simulink model "Bicycle_CTRA"  (R2018a)
settings: Solver=ode45  StartTime=0.0  StopTime=60  FixedStep=0.1  MaxStep=0.05  MinStep=1e-5  RelTol=1e-6  EnableMultiTasking=on
StopFcn:
  | run('CTRA_plotter.m');
model workspace (MAT data in the model file):
  B = 1.5289
  C = 1.0901
  D = 0.6
  E = -0.95084
  Iw = 1
  Iz = 1700
  Kphi_f = 57
  Kphi_r = 57
  hrc_f = 0
  hrc_r = 0
  hs = 0.56
  lf = 1
  lr = 1.6
  m = 1200
  re = 0.32
  tr = 1.5
undefined symbols (not defined in the file or in its folder): sigbuilder_block
libraries: commchan3 x6, simulink x1
settings Model: Creator=michaelstolz  LastModifiedBy=Mora
settings SolverCC: ZeroCrossControl=EnableAll  AutoInsertRateTranBlk=on  InsertRTBMode=Always
settings DataIOCC: SaveFormat=StructureWithTime  SignalLoggingSaveFormat=ModelDataLogs  SaveOutput=off  SignalLogging=off  SaveTime=off
settings OptimizationCC: LifeSpan=inf
settings DebuggingCC: UnderspecifiedInitializationDetection=Classic  MergeDetectMultiDrivingBlocksExec=none  SolverPrmCheckMsg=warning  FcnCallInpInsideContextMsg=warning  SFUnexpectedBacktrackingDiag=warning  SFNoUnconditionalDefaultTransitionDiag=warning  SFExecutionAtInitializationDiag=none
settings HardwareCC: ProdBitPerPointer=32  ProdBitPerSizeT=32  ProdBitPerPtrDiffT=32  ProdLargestAtomicFloat=None  ProdIntDivRoundTo=Undefined  ProdEndianess=Unspecified  ProdWordSize=32  ProdHWDeviceType=32-bit Generic
settings ModelReferenceCC: PropagateSignalLabelsOutOfModel=off
settings SFSimCC: SimParseCustomCode=off
settings CodeAppCC: StateflowObjectComments=on
settings GRTTargetCC: TargetLangStandard=C89/C90 (ANSI)  GeneratePreprocessorConditionals=Disable all
settings ConfigComp: CovMetricSettings=dw  CovHtmlReporting=on  CovSaveCumulativeToWorkspaceVar=on  CovSaveSingleToWorkspaceVar=on  CovExternalEMLEnable=off

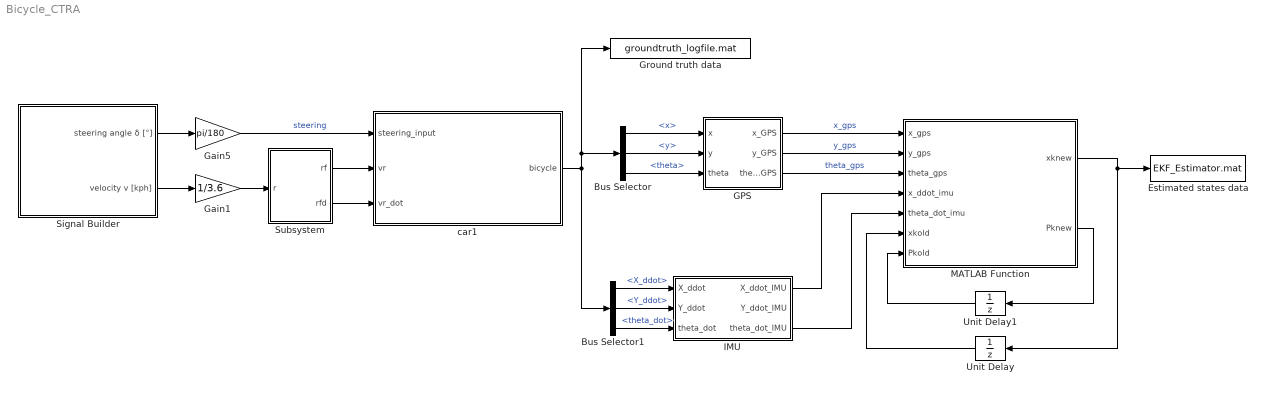
== system Bicycle_CTRA ==
  Bus Selector : BusSelector  OutputSignals=x,y,theta
  Bus Selector1 : BusSelector  OutputSignals=X_ddot,Y_ddot,theta_dot
  Estimated states data : ToFile  Filename=EKF_Estimator.mat  MatrixName=EKF  SaveFormat=Timeseries  SampleTime=1/50
  GPS : Subsystem
  Gain1 : Gain  Gain=1/3.6
  Gain5 : Gain  Gain=pi/180
  Ground truth data : ToFile  Filename=groundtruth_logfile.mat  MatrixName=GNDT  SaveFormat=Timeseries  SampleTime=1/50
  IMU : Subsystem
  MATLAB Function : MATLAB Function  TreatAsAtomicUnit=on
  Signal Builder : Subsystem  Tag=STV Subsys  LoadFcn=sigbuilder_block('load');  StartFcn=sigbuilder_block('start');  StopFcn=sigbuilder_block('stop');  ClipboardFcn=sigbuilder_block('clipboard');  mask(Sigbuilder block){tuvar=[0:10]}
      mask help: Simulink:masks:SigbuilderBlock_MD
      mask init:
      | if ~strcmp(get_param(bdroot(gcbh),'SimulationStatus'),'stopped') tuvar = sigbuilder_block('maskInit'); end
      settings: CopyFcn=sigbuilder_block('copy');  DeleteFcn=sigbuilder_block('delete');  ModelCloseFcn=sigbuilder_block('modelClose');  PreSaveFcn=sigbuilder_block('preSave');  PauseFcn=sigbuilder_block('pause');  ContinueFcn=sigbuilder_block('continue');  NameChangeFcn=sigbuilder_block('namechange');  OpenFcn=sigbuilder_block('open',[9 6 942 506.25 ]);  CloseFcn=sigbuilder_block('close');
      mask Display: plot(0, 0, 100, 100,[2, 2, 32, 32, 2], [68, 8, 8, 68, 68],[32, 2], [38, 38], [32, 19, 2],[53, 60, 44], [32, 17, 17, 2],[16, 16, 31, 31]);txt = getActiveGroup(gcbh);text(2, 100, txt,'verticalAlignment', 'top');
  Subsystem : Subsystem
  Unit Delay : UnitDelay  InitialCondition=[0, 0, 0.1, 1, 0.1, 0]'  SampleTime=-1
  Unit Delay1 : UnitDelay  InitialCondition=diag([1000000, 1000000, 10, 10, 10, 10],0)  SampleTime=-1
  car1 : Subsystem
  wires:
  Signal Builder/1(steering angle δ [°]) -> Gain5/1
  Signal Builder/2(velocity v [kph]) -> Gain1/1
  Gain5/1 -> car1/1(steering_input)  "steering"
  Subsystem/1(rf) -> car1/2(vr)
  car1/1(bicycle) -> Ground truth data/1, Bus Selector/1, Bus Selector1/1
  Bus Selector/1 -> GPS/1(x)  "<x>"
  Bus Selector/2 -> GPS/2(y)  "<y>"
  Gain1/1 -> Subsystem/1(r)
  Bus Selector/3 -> GPS/3(theta)  "<theta>"
  Subsystem/2(rfd) -> car1/3(vr_dot)
  Bus Selector1/1 -> IMU/1(X_ddot)  "<X_ddot>"
  Bus Selector1/2 -> IMU/2(Y_ddot)  "<Y_ddot>"
  Bus Selector1/3 -> IMU/3(theta_dot)  "<theta_dot>"
  GPS/1(x_GPS) -> MATLAB Function/1(x_gps)  "x_gps"
  GPS/2(y_GPS) -> MATLAB Function/2(y_gps)  "y_gps"
  GPS/3(theta_GPS) -> MATLAB Function/3(theta_gps)  "theta_gps"
  IMU/3(theta_dot_IMU) -> MATLAB Function/5(theta_dot_imu)
  MATLAB Function/2(Pknew) -> Unit Delay1/1
  MATLAB Function/1(xknew) -> Unit Delay/1, Estimated states data/1
  Unit Delay1/1 -> MATLAB Function/7(Pkold)
  Unit Delay/1 -> MATLAB Function/6(xkold)
  IMU/1(X_ddot_IMU) -> MATLAB Function/4(x_ddot_imu)

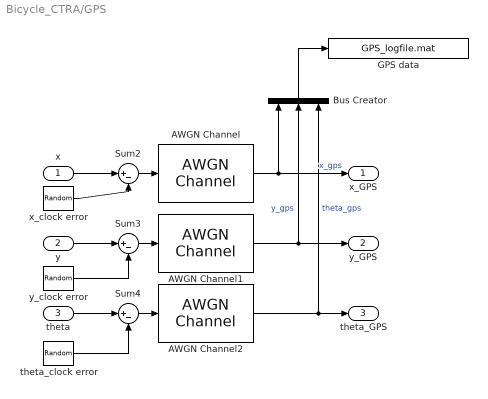
== system Bicycle_CTRA/GPS ==
  x : Inport
  y : Inport  Port=2
  theta : Inport  Port=3
  AWGN Channel : commchan3/AWGN Channel  InputProcessing=Columns as channels (frame based)  seed=40  noiseMode=Variance from mask  EbNodB=10  EsNodB=10  SNRdB=10  bitsPerSym=1  Ps=1  Tsym=1  variance=3
  AWGN Channel1 : commchan3/AWGN Channel  InputProcessing=Columns as channels (frame based)  seed=67  noiseMode=Variance from mask  EbNodB=10  EsNodB=10  SNRdB=10  bitsPerSym=1  Ps=1  Tsym=1  variance=3
  AWGN Channel2 : commchan3/AWGN Channel  InputProcessing=Columns as channels (frame based)  seed=67  noiseMode=Variance from mask  EbNodB=10  EsNodB=10  SNRdB=10  bitsPerSym=1  Ps=1  Tsym=1  variance=3/500
  Bus Creator : BusCreator  Inputs=3
  GPS data : ToFile  Filename=GPS_logfile.mat  MatrixName=GPS  SaveFormat=Timeseries  SampleTime=1/50
  Sum2 : Sum  Inputs=|+-
  Sum3 : Sum  Inputs=|+-
  Sum4 : Sum  Inputs=|+-
  theta_clock error : UniformRandomNumber  Minimum=0  Maximum=1e-9  SampleTime=3
  x_clock error : UniformRandomNumber  Minimum=0  Maximum=1e-9  SampleTime=3
  y_clock error : UniformRandomNumber  Minimum=0  Maximum=1e-9  SampleTime=3
  x_GPS : Outport
  y_GPS : Outport  Port=2
  theta_GPS : Outport  Port=3
  wires:
  AWGN Channel2/1 -> Bus Creator/3, theta_GPS/1  "theta_gps"
  x/1 -> Sum2/1
  Sum2/1 -> AWGN Channel/1
  Sum3/1 -> AWGN Channel1/1
  Sum4/1 -> AWGN Channel2/1
  y/1 -> Sum3/1
  y_clock error/1 -> Sum3/2
  AWGN Channel/1 -> Bus Creator/1, x_GPS/1  "x_gps"
  theta/1 -> Sum4/1
  AWGN Channel1/1 -> Bus Creator/2, y_GPS/1  "y_gps"
  x_clock error/1 -> Sum2/2
  theta_clock error/1 -> Sum4/2
  Bus Creator/1 -> GPS data/1

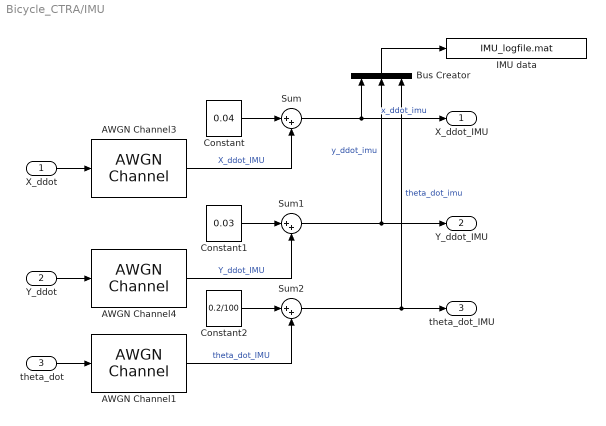
== system Bicycle_CTRA/IMU ==
  X_ddot : Inport
  Y_ddot : Inport  Port=2
  theta_dot : Inport  Port=3
  AWGN Channel1 : commchan3/AWGN Channel  InputProcessing=Columns as channels (frame based)  seed=67  noiseMode=Variance from mask  EbNodB=10  EsNodB=10  SNRdB=10  bitsPerSym=1  Ps=1  Tsym=1  variance=1/100
  AWGN Channel3 : commchan3/AWGN Channel  InputProcessing=Columns as channels (frame based)  seed=67  noiseMode=Variance from mask  EbNodB=10  EsNodB=10  SNRdB=10  bitsPerSym=1  Ps=1  Tsym=1  variance=0.08
  AWGN Channel4 : commchan3/AWGN Channel  InputProcessing=Columns as channels (frame based)  seed=67  noiseMode=Variance from mask  EbNodB=10  EsNodB=10  SNRdB=10  bitsPerSym=1  Ps=1  Tsym=1  variance=0.03
  Bus Creator : BusCreator  Inputs=3
  Constant : Constant  Value=0.04
  Constant1 : Constant  Value=0.03
  Constant2 : Constant  Value=0.2/100
  IMU data : ToFile  Filename=IMU_logfile.mat  MatrixName=IMU  SaveFormat=Timeseries  SampleTime=1/50
  Sum : Sum  Inputs=|++
  Sum1 : Sum  Inputs=|++
  Sum2 : Sum  Inputs=|++
  X_ddot_IMU : Outport
  Y_ddot_IMU : Outport  Port=2
  theta_dot_IMU : Outport  Port=3
  wires:
  X_ddot/1 -> AWGN Channel3/1
  Y_ddot/1 -> AWGN Channel4/1
  theta_dot/1 -> AWGN Channel1/1
  AWGN Channel3/1 -> Sum/2  "X_ddot_IMU"
  Sum/1 -> Bus Creator/1, X_ddot_IMU/1  "x_ddot_imu"
  Constant/1 -> Sum/1
  Constant1/1 -> Sum1/1
  Sum1/1 -> Bus Creator/2, Y_ddot_IMU/1  "y_ddot_imu"
  AWGN Channel4/1 -> Sum1/2  "Y_ddot_IMU"
  Constant2/1 -> Sum2/1
  Sum2/1 -> Bus Creator/3, theta_dot_IMU/1  "theta_dot_imu"
  AWGN Channel1/1 -> Sum2/2  "theta_dot_IMU"
  Bus Creator/1 -> IMU data/1

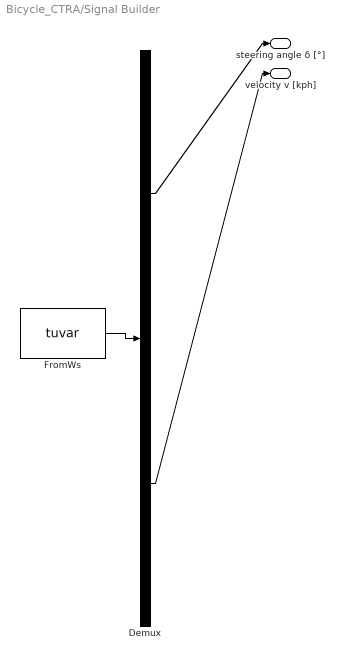
== system Bicycle_CTRA/Signal Builder ==
  Demux : Demux  Tag=STV Demux  Outputs=2
  FromWs : FromWorkspace  Tag=STV FromWs  VariableName=tuvar  SampleTime=0
      SigBuilderData=|
      | common.afterFinalStr = 'Extrapolate'
      | common.sampleTime = 0
      | dataSet(1).timeRange = [0 20]
      | dataSet(1).name = 'Line'
      | dataSet(2).timeRange = [0 20]
      | dataSet(2).name = 'Left curve'
      | dataSet(3).timeRange = [0 60]
      | dataSet(3).name = 'Line Curves'
      | sbobj.Groups(1).Name = 'Line'
      | sbobj.Groups(1).Signals(1).Name = 'steering angle δ [°]'
      | sbobj.Groups(1).Signals(1).XData = [0 20]
      | sbobj.Groups(1).Signals(1).YData = [0 0]
      | sbobj.Groups(1).Signals(2).Name = 'velocity v [kph]'
      | sbobj.Groups(1).Signals(2).XData = [0 6 15 20]
      | sbobj.Groups(1).Signals(2).YData = [0 100 150 150]
      | sbobj.Groups(1).TimeRange = [0 20]
      | sbobj.Groups(2).Name = 'Left curve'
      | sbobj.Groups(2).Signals(1).Name = 'steering angle δ [°]'
      | sbobj.Groups(2).Signals(1).XData = [0 20]
      | sbobj.Groups(2).Signals(1).YData = [3.61 3.61]
      | sbobj.Groups(2).Signals(2).Name = 'velocity v [kph]'
      | sbobj.Groups(2).Signals(2).XData = [0 10 20]
      | sbobj.Groups(2).Signals(2).YData = [0 79.5 80]
      | sbobj.Groups(2).TimeRange = [0 20]
      | sbobj.Groups(3).Name = 'Line Curves'
      | sbobj.Groups(3).Signals(1).Name = 'steering angle δ [°]'
      | sbobj.Groups(3).Signals(1).XData = [0 15 25 30 40 40 52 54 60]
      | sbobj.Groups(3).Signals(1).YData = [0 0 -2 -2 2 1.98 2 0 0]
      | sbobj.Groups(3).Signals(2).Name = 'velocity v [kph]'
      | sbobj.Groups(3).Signals(2).XData = [0 15 30 35 40 50 60]
      | sbobj.Groups(3).Signals(2).YData = [0 100 60 40 60 60 60]
      | sbobj.Groups(3).TimeRange = [0 60]
  steering angle δ [°] : Outport  Tag=STV Outport
  velocity v [kph] : Outport  Tag=STV Outport  Port=2
  wires:
  FromWs/1 -> Demux/1
  Demux/1 -> steering angle δ [°]/1
  Demux/2 -> velocity v [kph]/1

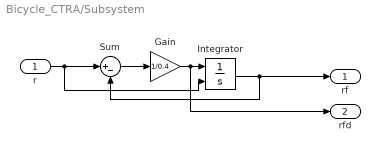
== system Bicycle_CTRA/Subsystem ==
  r : Inport
  Gain : Gain  Gain=1/0.4
  Integrator : Integrator  InitialConditionSource=external
  Sum : Sum  Inputs=|+-
  rf : Outport
  rfd : Outport  Port=2
  wires:
  Gain/1 -> rfd/1, Integrator/1
  Sum/1 -> Gain/1
  Integrator/1 -> rf/1, Sum/2
  r/1 -> Integrator/2, Sum/1

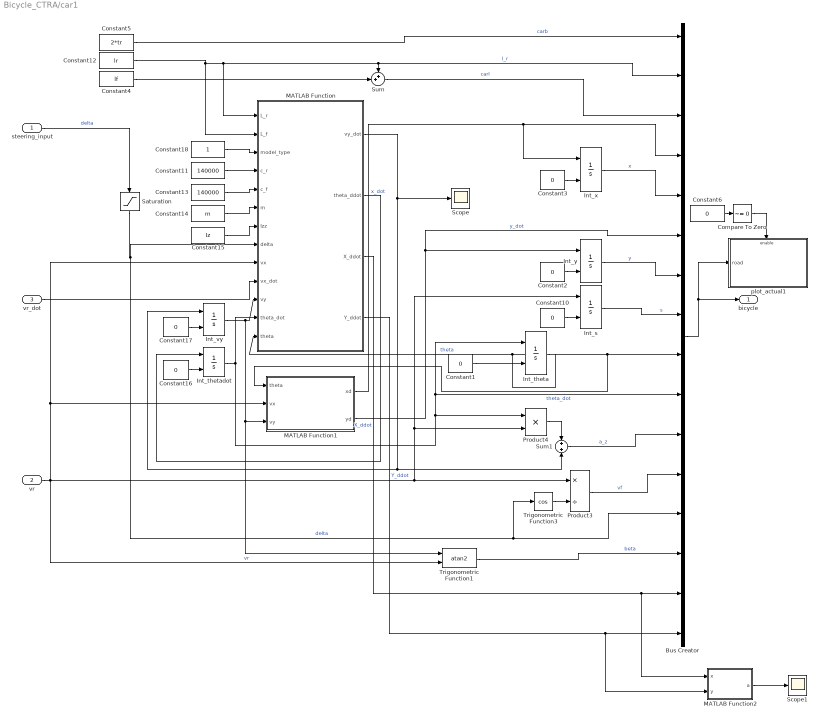
== system Bicycle_CTRA/car1 ==
  steering_input : Inport
  vr : Inport  Port=2
  vr_dot : Inport  Port=3
  Bus Creator : BusCreator  Inputs=16
  Compare To Zero : simulink/Logic and Bit Operations/Compare To Zero  relop=~=  OutDataTypeStr=boolean
  Constant{1..3,6,10,16..17} (7 alike) : Constant  Value=0
  Constant11 : Constant  Value=140000
  Constant12 : Constant  Value=lr
  Constant13 : Constant  Value=140000
  Constant14 : Constant  Value=m
  Constant15 : Constant  Value=Iz
  Constant18 : Constant
  Constant4 : Constant  Value=lf
  Constant5 : Constant  Value=2*tr
  Int_s : Integrator  InitialConditionSource=external
  Int_theta : Integrator  InitialConditionSource=external
  Int_thetadot : Integrator  InitialConditionSource=external
  Int_vy : Integrator  InitialConditionSource=external
  Int_x : Integrator  InitialConditionSource=external
  Int_y : Integrator  InitialConditionSource=external
  MATLAB Function : MATLAB Function  TreatAsAtomicUnit=on
  MATLAB Function1 : MATLAB Function  TreatAsAtomicUnit=on
  MATLAB Function2 : MATLAB Function  TreatAsAtomicUnit=on
  Product3 : Product  Inputs=*/
  Product4 : Product
  Saturation : Saturate  UpperLimit=pi/8  LowerLimit=-pi/8
  Scope : Scope
  Scope1 : Scope
  Sum : Sum  Inputs=++|
  Sum1 : Sum  Inputs=+|+
  Trigonometric Function1 : Trigonometry  Operator=atan2
  Trigonometric Function3 : Trigonometry  Operator=cos
  plot_actual1 : Subsystem  mask{dt=0.1}
      mask prompts: dt "Sample rate for plotting"
      mask Display:
      | text(.2,.8,'\fontname{palatino}\fontsize{15}\bf plot car',...
      |       'HorizontalAlignment','left','texmode','on');
      | text(.25,.5,['\fontname{palatino}\fontsize{10}rate = ',sprintf('%4.2f[s]',dt)],...
      |       'HorizontalAlignment','left','texmode','on');
  bicycle : Outport
  wires:
  Saturation/1 -> MATLAB Function/8(delta), Bus Creator/13, Trigonometric Function3/1  "delta"
  Int_vy/1 -> MATLAB Function/11(vy), MATLAB Function1/3(vy), Trigonometric Function1/1
  Trigonometric Function1/1 -> Bus Creator/14  "beta"
  Constant18/1 -> MATLAB Function/3(model_type)
  MATLAB Function/1(vy_dot) -> Scope/1, Int_vy/1, Sum1/2
  Product4/1 -> Sum1/1
  Constant17/1 -> Int_vy/2
  Constant16/1 -> Int_thetadot/2
  MATLAB Function/2(theta_ddot) -> Int_thetadot/1
  Constant15/1 -> MATLAB Function/7(Izz)
  Constant14/1 -> MATLAB Function/6(m)
  Constant13/1 -> MATLAB Function/5(c_f)
  Constant11/1 -> MATLAB Function/4(c_r)
  Constant12/1 -> Sum/1, Bus Creator/2, MATLAB Function/1(L_r), MATLAB Function/2(L_f)  "l_r"
  Constant4/1 -> Sum/2
  Sum1/1 -> Bus Creator/11  "a_z"
  Constant3/1 -> Int_x/2
  Constant2/1 -> Int_y/2
  Constant1/1 -> Int_theta/2
  Bus Creator/1 -> plot_actual1/1(road), bicycle/1
  Int_x/1 -> Bus Creator/5  "x"
  Int_y/1 -> Bus Creator/7  "y"
  MATLAB Function1/1(xd) -> Bus Creator/4, Int_x/1  "x_dot"
  MATLAB Function1/2(yd) -> Int_y/1, Bus Creator/6  "y_dot"
  Int_theta/1 -> Bus Creator/9, MATLAB Function1/1(theta), MATLAB Function/13(theta)  "theta"
  vr/1 -> Trigonometric Function1/2, Product4/2, Int_s/1, Product3/1, MATLAB Function1/2(vx), MATLAB Function/9(vx)  "vr"
  Sum/1 -> Bus Creator/3  "carl"
  Constant5/1 -> Bus Creator/1  "carb"
  Int_thetadot/1 -> MATLAB Function/12(theta_dot), Product4/1, Int_theta/1, Bus Creator/10  "theta_dot"
  Trigonometric Function3/1 -> Product3/2
  Product3/1 -> Bus Creator/12  "vf"
  Compare To Zero/1 -> plot_actual1/Enable
  Constant6/1 -> Compare To Zero/1
  steering_input/1 -> Saturation/1  "delta"
  Int_s/1 -> Bus Creator/8  "s"
  Constant10/1 -> Int_s/2
  vr_dot/1 -> MATLAB Function/10(vx_dot)
  MATLAB Function/3(X_ddot) -> MATLAB Function2/1(x), Bus Creator/15  "X_ddot"
  MATLAB Function/4(Y_ddot) -> MATLAB Function2/2(y), Bus Creator/16  "Y_ddot"
  MATLAB Function2/1(a) -> Scope1/1

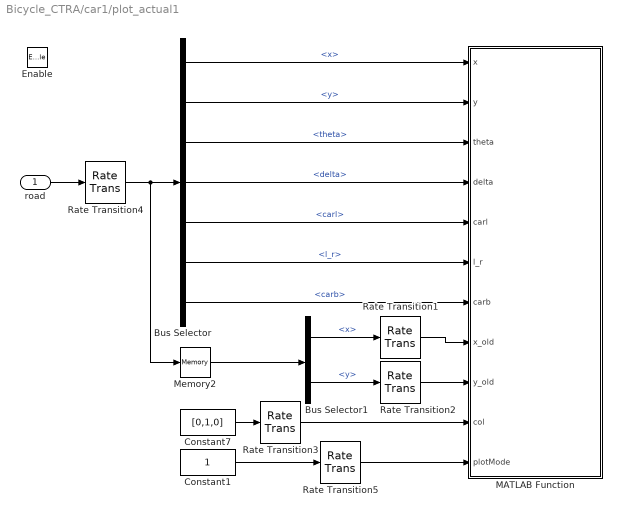
== system Bicycle_CTRA/car1/plot_actual1 ==
  road : Inport
  Enable : EnablePort
  Bus Selector : BusSelector  OutputSignals=x,y,theta,delta,carl,l_r,carb
  Bus Selector1 : BusSelector  OutputSignals=x,y
  Constant1 : Constant
  Constant7 : Constant  Value=[0,1,0]
  MATLAB Function : MATLAB Function  TreatAsAtomicUnit=on
  Memory2 : Memory
  Rate Transition{1..5} (5 alike) : RateTransition  OutPortSampleTime=dt
  wires:
  Rate Transition5/1 -> MATLAB Function/11(plotMode)
  Constant1/1 -> Rate Transition5/1
  Bus Selector/6 -> MATLAB Function/6(l_r)  "<l_r>"
  Bus Selector/3 -> MATLAB Function/3(theta)  "<theta>"
  Bus Selector1/2 -> Rate Transition2/1  "<y>"
  Bus Selector1/1 -> Rate Transition1/1  "<x>"
  Memory2/1 -> Bus Selector1/1
  Rate Transition4/1 -> Bus Selector/1, Memory2/1
  Bus Selector/1 -> MATLAB Function/1(x)  "<x>"
  Bus Selector/2 -> MATLAB Function/2(y)  "<y>"
  road/1 -> Rate Transition4/1
  Bus Selector/7 -> MATLAB Function/7(carb)  "<carb>"
  Bus Selector/5 -> MATLAB Function/5(carl)  "<carl>"
  Rate Transition1/1 -> MATLAB Function/8(x_old)
  Rate Transition2/1 -> MATLAB Function/9(y_old)
  Bus Selector/4 -> MATLAB Function/4(delta)  "<delta>"
  Constant7/1 -> Rate Transition3/1
  Rate Transition3/1 -> MATLAB Function/10(col)

== matlab function Bicycle_CTRA/car1/MATLAB Function ==
  data: L_r input; vy_dot output; L_f input; model_type input; c_r input; c_f input; m input; Izz input; delta input; vx input; vx_dot input; vy input; theta_dot input; theta_ddot output; X_ddot output; Y_ddot output; theta input
function [ vy_dot, theta_ddot, X_ddot, Y_ddot] = dynCar(L_r, L_f, model_type, c_r, c_f, m,...
                                       Izz, delta, vx, vx_dot, vy, theta_dot, theta)
%#codegen
if abs(vx) < 0.01
    model_type=0;
end

switch model_type
    case 1 % linearized Model   
        A = [ -(c_f+c_r)/(vx*m),  (-c_f*L_f+c_r*L_r)/(vx*m) - vx;...
               (-c_f*L_f+c_r*L_r)/(Izz*vx), -(c_r*L_r^2+c_f*L_f^2)/(Izz*vx)];
        
        vy_dot     = A(1,:)*[vy; theta_dot] +  c_f/m *delta;
        theta_ddot = A(2,:)*[vy; theta_dot] +  c_f*L_f/Izz * delta;
        
    otherwise % nonlinear Model
        a_r = - atan2(vy-L_r*theta_dot, vx);
        a_f = delta - atan2(vy+L_f*theta_dot,vx);
        
        vy_dot     = 1/m   * (c_f*a_f*cos(delta)     + c_r*a_r ) - theta_dot*vx;
        theta_ddot = 1/Izz * (c_f*a_f*L_f*cos(delta) - c_r*L_r*a_r);
end

% Global accelerations

%X_ddot     = vx_dot - vy * theta_dot;
X_ddot     = vx_dot;
Y_ddot     = vy_dot + vx * theta_dot;
end

== matlab function Bicycle_CTRA/car1/MATLAB Function1 ==
  data: theta input; xd output; yd output; vx input; vy input
function [ xd, yd] = dynCar( theta,vx, vy )
%#codegen

R = [cos(theta), -sin(theta); sin(theta), cos(theta)];
xd = R(1,:)*[vx;vy];
yd = R(2,:)*[vx;vy];
end

== matlab function Bicycle_CTRA/MATLAB Function ==
  data: x_gps input; xknew output; y_gps input; theta_gps input; x_ddot_imu input; theta_dot_imu input; Pknew output; xkold input; Pkold input
function [xknew, Pknew] = EKF(x_gps, y_gps, theta_gps, x_ddot_imu, theta_dot_imu, xkold, Pkold)

close all

%Sampling time T for f = 50 Hz
T = 1/50; 

%Assigning states using state vector
x = xkold(1);
y = xkold(2);
theta = xkold(3);
v = xkold(4);
theta_dot = xkold(5);
a = xkold(6);


%Measurement vector [z]
%z = [x_gps y_gps theta_gps x_ddot_imu y_ddot_imu theta_dot_imu]';
z = [x_gps y_gps theta_gps x_ddot_imu theta_dot_imu]';

%Process noise covariance matrix [Q]
nu_a     = 2; %m/s^2
nu_theta = 0.1; % rad/s

%standard deviations
std_x         = (1/6)* T^3 * nu_a;
std_theta     = 0.5 * T^2 * nu_theta;
std_v         = 0.5 * T^2 * nu_a;
std_thetaddot = T * nu_theta;
std_a         = T * nu_a;


Q = diag([std_x^2, std_x^2, std_theta^2, std_v^2, std_thetaddot^2, std_a^2],0);

%Q = diag([7.6e-4,7.6e-4,5e-6,8e-2,8e-2,1e-5],0);

%Sensors noise covariance matrix [R]


%R = diag([3, 3, 3/500, 0.093, 0.15, 1/100],0);
R = diag([3, 3, 3/500, 0.08, 1/100],0);


%State Transition matrix Definition ([f] non-linear matrix, [A] Jacobian linear matrix) 
model_type = 0;

if theta_dot == 0 
    model_type=1;
end

switch model_type
    case 1 % straight-line driving case   
        f =[v*T*cos(theta) + a*(T^2/2)*cos(theta) + x;
            v*T*sin(theta) + a*(T^2/2)*sin(theta) + y;
            theta_dot*T + theta;
            a*T + v;
            theta_dot;
            a];

        A =[1, 0, (-v*T-a*(T^2/2))*sin(theta), 0, 0, 0;
            0, 1,  (v*T+a*(T^2/2))*cos(theta), 0, 0, 0;
            0, 0, 1, 0, T, 0;
            0, 0, 0, 1, 0, T;
            0, 0, 0, 0, 1, 0;
            0, 0, 0, 0, 0, 1];
            
        
    otherwise % non-straight line driving
        f =[1/theta_dot^2*(-v*theta_dot*sin(theta)-a*cos(theta)+theta_dot*(v+a*T)*sin(theta+theta_dot*T)...
            +a*cos(theta+theta_dot*T))+x;
            1/theta_dot^2*(-a*sin(theta)+v*theta_dot*cos(theta)+a*sin(theta+theta_dot*T)...
            -theta_dot*(v+a*T)*cos(theta+theta_dot*T))+y;
            theta_dot*T + theta;
            a*T + v;
            theta_dot;
            a];
            
            

        A =[1, 0, 1/theta_dot^2*(a*sin(theta)-v*theta_dot*cos(theta)-a*sin(theta+theta_dot*T)+...
            theta_dot*(v+a*T)*cos(theta+theta_dot*T)), 1/theta_dot*(-sin(theta)+sin(theta+theta_dot*T)),...
            1/theta_dot^3*(v*theta_dot*sin(theta)+2*a*cos(theta)+(-theta_dot*v-2*a*theta_dot*T)*... %b1
            sin(theta+theta_dot*T)+(-2*a+theta_dot^2*T*(v+a*T))*cos(theta+theta_dot*T)), ...        %b1
            1/theta_dot^2*(-cos(theta)+theta_dot*T*sin(theta+theta_dot*T)+cos(theta+theta_dot*T));  %row1
            0, 1, 1/theta_dot^2*(-a*cos(theta)-v*theta_dot*sin(theta)+a*cos(theta+theta_dot*T)+...
            theta_dot*(v+a*T)*sin(theta+theta_dot*T)), 1/theta_dot*(cos(theta)-cos(theta+theta_dot*T)),...
            1/theta_dot^3*(2*a*sin(theta)-v*theta_dot*cos(theta)+(-2*a+theta_dot^2*T*(v+a*T))*...   %b2
            sin(theta+theta_dot*T)+(theta_dot*v+2*a*theta_dot*T)*cos(theta+theta_dot*T)),...        %b2
            1/theta_dot^2*(-sin(theta)+sin(theta+theta_dot*T)-theta_dot*T*cos(theta+theta_dot*T));  %row2
            0, 0, 1, 0, T, 0;
            0, 0, 0, 1, 0, T;
            0, 0, 0, 0, 1, 0;
            0, 0, 0, 0, 0, 1];
end

%Prediction step
xknewp = f; 
Pknewp = A*Pkold*A'+Q;

% Measurement model
% Measurement non-linear vector h(x)
% h = [xknewp(1) xknewp(2) xknewp(3) xknewp(6)*cos(xknewp(3)) xknewp(6)*sin(xknewp(3)) xknewp(5)]';

% Measurement Jacobian matrix [H]
H = [1 0 0 0 0 0;
     0 1 0 0 0 0;
     0 0 1 0 0 0;
     0 0 0 0 0 1
     0 0 0 0 1 0];
 
% H = [1 0 0 0 0 0;
%      0 1 0 0 0 0;
%      0 0 1 0 0 0;
%      0 0 -xknewp(6)*sin(xknewp(3)) 0 0 cos(xknewp(3));
%      0 0  xknewp(6)*cos(xknewp(3)) 0 0 sin(xknewp(3));
%      0 0 0 0 1 0];
     

%Estimation step
Y = z - H*xknewp;
S = H * Pknewp * H' + R;
K = Pknewp * H' /S;
xknew = xknewp + K*Y;
Pknew = Pknewp - K*H*Pknewp;
end

== matlab function Bicycle_CTRA/car1/plot_actual1/MATLAB Function ==
  data: x input; y input; theta input; delta input; carl input; l_r input; carb input; x_old input; y_old input; col input; plotMode input
function fcn( x, y, theta,delta,carl,l_r, carb, x_old, y_old, col, plotMode)
%#codegen
coder.extrinsic('delete');
fh = figure(1);
hold on; box on; grid on;
xlim([x-100,x+100]);
ylim([y-100,y+100]);
axis equal

R    = [ cos(theta), -sin(theta);...
         sin(theta), cos(theta)];   
           
plot([x_old,x],[y_old,y],'Color',col);
plot(x,y,'.','Color',col);
         
carx = [-l_r, carl-l_r, carl-l_r, -l_r, -l_r];
cary = [-carb, -carb, carb, carb, -carb]*0.5;
carxn = R(1,:)*[carx;cary];
caryn = R(2,:)*[carx;cary];

if plotMode==1,
  delete(findall(fh,'Tag', 'vehicle'));  
end

plot(carxn+x,caryn+y,'-','Color',col,'Tag', 'vehicle');

Rd    = [ cos(delta), -sin(delta);...
         sin(delta), cos(delta)]*R; 

for w=1:4
   wheelcx = [carx(w),carx(w)];
   wheelcy = [cary(w),cary(w)];
   wheelwx = [-carl carl]*0.25;
   wheelwy = [0 0];
      
   wheelcxn =  R(1,:)*[wheelcx;wheelcy];
   wheelcyn =  R(2,:)*[wheelcx;wheelcy];
   if w==2 || w==3,
       wheelwxn =  Rd(1,:)*[wheelwx;wheelwy];
       wheelwyn =  Rd(2,:)*[wheelwx;wheelwy];
   else
       wheelwxn =  R(1,:)*[wheelwx;wheelwy];
       wheelwyn =  R(2,:)*[wheelwx;wheelwy];
   end
   plot(wheelcxn+[x,x]+wheelwxn,wheelcyn+[y,y]+wheelwyn,...
       '-k', 'linewidth',2,'Tag', 'vehicle');
end


end

== matlab function Bicycle_CTRA/car1/MATLAB Function2 ==
  data: x input; a output; y input
function a = fcn(x,y)

a = sqrt(x^2+y^2);

end
